simulink model "FINAL_FULL_CONTROLLER"  (R2023b)
settings: Solver=VariableStepAuto  StartTime=0.0  StopTime=10  MaxStep=1e-2  RelTol=1e-6
values from neighbouring files (symbols this model uses):
  cq = -rho*(pi*re^2)*(re^2)*Cq    (= -5.82688103164e-07)    [PARAMETRI_DRONE.m]
  Cq = 0.002508    [PARAMETRI_DRONE.m]
  ct = rho*(pi*re^2)*(re^2)*Ct    (= 3.66666014519e-06)    [PARAMETRI_DRONE.m]
  Ct = 0.015782    [PARAMETRI_DRONE.m]
  dx = 0.035/(2*sqrt(2))    [PARAMETRI_DRONE.m]
  dy = 0.035/(2*sqrt(2))    [PARAMETRI_DRONE.m]
  g = 9.81    [PARAMETRI_DRONE.m]
  I = Inertial_Matrix_DART(m1, m2, m3, m4, m, d1, d2, d3, d4, d5, dx, dy, r, h, a1, b1, c1, a2, b2, c2, a3, b3, c3, a4, b4, c4)    [PARAMETRI_DRONE.m]
  m = 0.055    [PARAMETRI_DRONE.m]
  m1 = 0.135    [PARAMETRI_DRONE.m]
  m2 = 0.602    [PARAMETRI_DRONE.m]
  m3 = 0.228    [PARAMETRI_DRONE.m]
  m4 = 0.055    [PARAMETRI_DRONE.m]
  re = 0.0889    [PARAMETRI_DRONE.m]
  wmax = RPMmax*(2*pi)/60    (= 2350.85378268)    [PARAMETRI_DRONE.m]
libraries: slpidlib x9, simulink x4, shared6dof x1, aerolibpropulsion2 x1, dspinverses x1
(part 2 of 2)

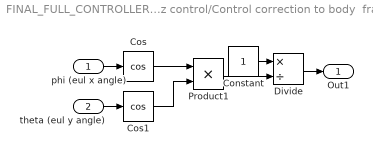
== system FINAL_FULL_CONTROLLER/ALTITUDE CONTOL/Vz control/Control correction to body  frame ==
  phi (eul x angle) : Inport
  theta (eul y angle) : Inport  Port=2
  Constant : Constant
  Cos : Trigonometry  Operator=cos
  Cos1 : Trigonometry  Operator=cos
  Divide : Product  Inputs=*/
  Product1 : Product
  Out1 : Outport
  wires:
  theta (eul y angle)/1 -> Cos1/1
  phi (eul x angle)/1 -> Cos/1
  Product1/1 -> Divide/2
  Constant/1 -> Divide/1
  Divide/1 -> Out1/1
  Cos1/1 -> Product1/2
  Cos/1 -> Product1/1
